simulink subsystem "PieroO"  (R2025a)
settings: Solver=VariableStepAuto  StartTime=0.0  StopTime=10.0  RelTol=1e-3
settings Model: Creator=Antonio  LastModifiedBy=aj
settings RTWCC: GPUComputeCapability=3.5

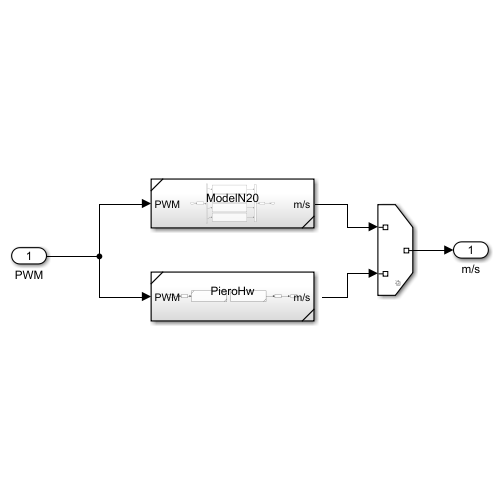
[thumbnail: Simulink's stored preview of the top-level diagram]
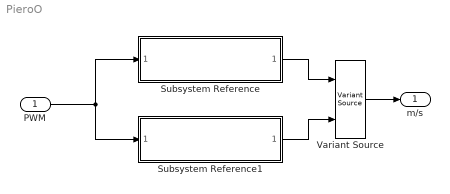
== system PieroO ==
  PWM : Inport
  Subsystem Reference : Subsystem  ReferencedSubsystem=ModelN20
  Subsystem Reference1 : Subsystem  ReferencedSubsystem=PieroHw
  Variant Source : VariantSource  VariantControlMode=sim codegen switching  VariantControls={(sim), (codegen)}
  m/s : Outport
  wires:
  PWM/1 -> Subsystem Reference/1, Subsystem Reference1/1
  Variant Source/1 -> m/s/1
  Subsystem Reference/1 -> Variant Source/1
  Subsystem Reference1/1 -> Variant Source/2
